simulink model "IFDA_5_2_Test1_Simulink"  (R2025b)
settings: Solver=VariableStepAuto  StartTime=0.0  StopTime=700  RelTol=1e-3
values from neighbouring files (symbols this model uses):
  lambda0 = zeros(6,1)    [IFDA_5_2_Test1.m]
  z0 = zeros(6,1)    [IFDA_5_2_Test1.m]
settings Model: Creator=ShuochengTian  LastModifiedBy=ShuochengTian
settings DataIOCC: ReturnWorkspaceOutputs=off

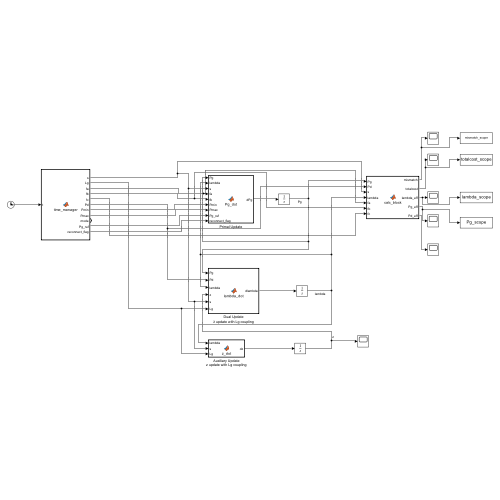
[thumbnail: Simulink's stored preview of the top-level diagram]
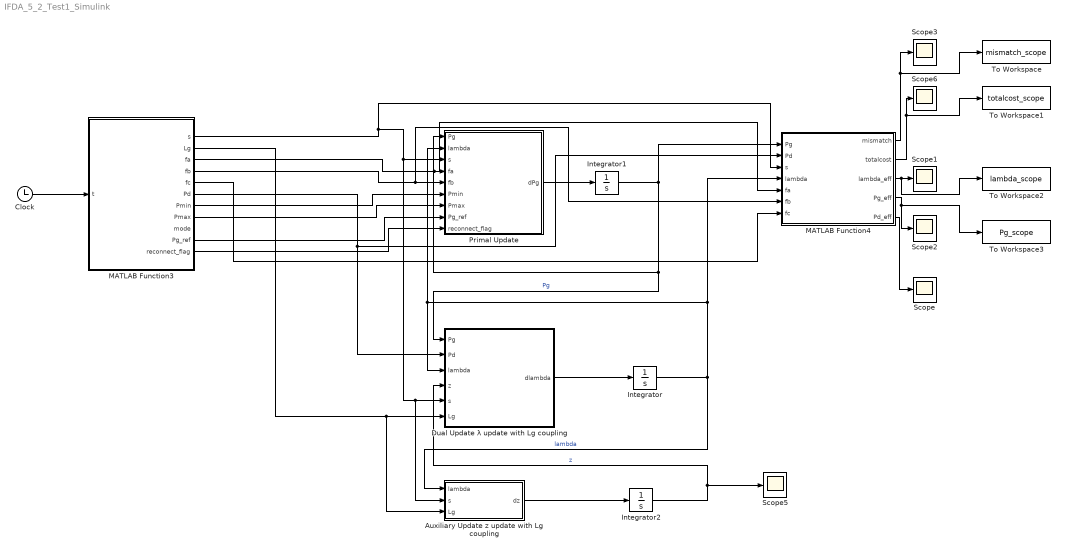
== system IFDA_5_2_Test1_Simulink ==
  Auxiliary Update z update with Lg coupling : MATLAB Function  TreatAsAtomicUnit=on
  Clock : Clock
  Dual Update λ update with Lg coupling : MATLAB Function  TreatAsAtomicUnit=on
  Integrator : Integrator  InitialCondition=lambda0
  Integrator1 : Integrator  InitialCondition=[0;0;0;0;0;0]
  Integrator2 : Integrator  InitialCondition=z0
  MATLAB Function3 : MATLAB Function  TreatAsAtomicUnit=on
  MATLAB Function4 : MATLAB Function  TreatAsAtomicUnit=on
  Primal Update : MATLAB Function  TreatAsAtomicUnit=on
  Scope{,1..3,5..6} (6 alike) : Scope
      Scope settings: ActiveDisplayYMinimum=-1  ActiveDisplayYMaximum=1
      Scope1 settings: ActiveDisplayYMinimum=-65.150992520934949  ActiveDisplayYMaximum=108.34326457907353
      Scope2 settings: ActiveDisplayYMinimum=-20.980945612997647  ActiveDisplayYMaximum=188.82851051697887  DataLoggingVariableName=Pg_scope
      Scope3 settings: ActiveDisplayYMinimum=-491.25638356925219  ActiveDisplayYMaximum=557.32192082133315  DataLoggingVariableName=ScopeData3
      Scope5 settings: ActiveDisplayYMinimum=-43.668129807631672  ActiveDisplayYMaximum=39.234905001957  DataLoggingVariableName=ScopeData5
      Scope6 settings: ActiveDisplayYMinimum=-1090.2784061772797  ActiveDisplayYMaximum=14121.754852896567  DataLoggingVariableName=ScopeData6
  To Workspace : ToWorkspace  VariableName=mismatch_scope  SaveFormat=Structure With Time  SampleTime=-1
  To Workspace1 : ToWorkspace  VariableName=totalcost_scope  SaveFormat=Structure With Time  SampleTime=-1
  To Workspace2 : ToWorkspace  VariableName=lambda_scope  SaveFormat=Structure With Time  SampleTime=-1
  To Workspace3 : ToWorkspace  VariableName=Pg_scope  SaveFormat=Structure With Time  SampleTime=-1
  wires:
  Integrator1/1 -> Primal Update/1(Pg), Dual Update λ update with Lg coupling/1(Pg), MATLAB Function4/1(Pg)  "Pg"
  Integrator2/1 -> Scope5/1, Dual Update λ update with Lg coupling/4(z)  "z"
  Auxiliary Update z update with Lg coupling/1(dz) -> Integrator2/1
  Integrator/1 -> MATLAB Function4/4(lambda), Dual Update λ update with Lg coupling/3(lambda), Primal Update/2(lambda), Auxiliary Update z update with Lg coupling/1(lambda)  "lambda"
  Primal Update/1(dPg) -> Integrator1/1
  MATLAB Function3/6(Pd) -> Dual Update λ update with Lg coupling/2(Pd), MATLAB Function4/2(Pd)
  Dual Update λ update with Lg coupling/1(dlambda) -> Integrator/1
  Clock/1 -> MATLAB Function3/1(t)
  MATLAB Function3/1(s) -> MATLAB Function4/3(s), Auxiliary Update z update with Lg coupling/2(s), Dual Update λ update with Lg coupling/5(s), Primal Update/3(s)
  MATLAB Function3/2(Lg) -> Dual Update λ update with Lg coupling/6(Lg), Auxiliary Update z update with Lg coupling/3(Lg)
  MATLAB Function3/3(fa) -> MATLAB Function4/5(fa), Primal Update/4(fa)
  MATLAB Function3/4(fb) -> Primal Update/5(fb), MATLAB Function4/6(fb)
  MATLAB Function3/7(Pmin) -> Primal Update/6(Pmin)
  MATLAB Function3/8(Pmax) -> Primal Update/7(Pmax)
  MATLAB Function3/10(Pg_ref) -> Primal Update/8(Pg_ref)
  MATLAB Function3/11(reconnect_flag) -> Primal Update/9(reconnect_flag)
  MATLAB Function4/1(mismatch) -> To Workspace/1, Scope3/1
  MATLAB Function4/4(Pg_eff) -> Scope2/1, To Workspace3/1
  MATLAB Function4/2(totalcost) -> To Workspace1/1, Scope6/1
  MATLAB Function3/5(fc) -> MATLAB Function4/7(fc)
  MATLAB Function4/5(Pd_eff) -> Scope/1
  MATLAB Function4/3(lambda_eff) -> To Workspace2/1, Scope1/1

== matlab function IFDA_5_2_Test1_Simulink/Dual Update λ update with Lg coupling ==
  data: Pg input; Pd input; dlambda output; lambda input; z input; s input; Lg input
function dlambda = lambda_dot(Pg, Pd, lambda, z, s, Lg)

n = 6;
dlambda = zeros(n,1);
%实际参与系统供需平衡的发电功率

Pg_eff = s .* Pg;
Pd_eff = s .* Pd;

%按资源分配算法计算原始

dlambda_raw = -Lg * lambda - Lg * z + (Pd_eff - Pg_eff);
%dlambda = dlambda_raw;

%对离线节点可选择冻结
for i = 1:n
   if s(i) == 0
       dlambda(i) = 0;
   else
       dlambda(i) = dlambda_raw(i);
   end
end

== matlab function IFDA_5_2_Test1_Simulink/Primal Update ==
  data: Pg input; lambda input; s input; fa input; fb input; Pmin input; Pmax input; Pg_ref input; dPg output; reconnect_flag input
function dPg = Pg_dot(Pg, lambda, s, fa, fb, Pmin, Pmax, Pg_ref, reconnect_flag)

n = 6;
dPg = zeros(n,1);
kr = 50;

for i = 1:n
    %% 若机组离线，直接冻结
    if s(i) == 0
        dPg(i) = 0;
        
    %% 若机组处于恢复过渡阶段
    elseif reconnect_flag(i) == 1
        v_i = kr * (Pg_ref(i) - Pg(i));
        if (Pg(i) <= Pmin(i)) && (v_i < 0)
            dPg(i) = 0;
        elseif (Pg(i) >= Pmax(i)) && (v_i > 0)
            dPg(i) = 0;
        else
            dPg(i) = v_i;
        end
        
    %% 正常在线运行：按原投影动态
    else
        
        grad_i = 2*fa(i)*Pg(i) + fb(i);
        
        
        v_i = -grad_i + lambda(i);
        
        if (Pg(i) <= Pmin(i)) && (v_i < 0)
            dPg(i) = 0;
        elseif (Pg(i) >= Pmax(i)) && (v_i > 0)
            dPg(i) = 0;
        else
            dPg(i) = v_i;
        end
    end
end

== matlab function IFDA_5_2_Test1_Simulink/Auxiliary Update z update with Lg coupling ==
  data: lambda input; dz output; s input; Lg input
function dz = z_dot(lambda, s, Lg)

n = 6;
dz = zeros(n,1);


% 先计算原始动态
dz_raw = Lg * lambda;
%dz = dz_raw;


% 对离线节点冻结
for i = 1:n
    if s(i) == 0
        dz(i) = 0;
    else
        dz(i) = dz_raw(i);
    end
end

== matlab function IFDA_5_2_Test1_Simulink/MATLAB Function3 ==
  data: t input; s output; Lg output; fa output; fb output; fc output; Pd output; Pmin output; Pmax output; mode output; Pg_ref output; reconnect_flag output
function [s,Lg,fa,fb,fc,Pd,Pmin,Pmax,mode,Pg_ref,reconnect_flag] = time_manager(t)
%% 断开前的旧配置
a_pre = [0.0100; 0.0250; 0.0200; 0.0090; 0.0180; 0.0340];

b_pre = [10.5;   12.0;   15.0;   11.5;   13.0;   9.5];

c_pre = [20; 25; 30; 22; 28; 18];

Pd_pre = [90; 80; 70; 85; 60; 55];

Pmin_pre = [20; 25; 15; 30; 18; 12];

Pmax_pre = [180; 200; 160; 220; 170; 150];

%% 恢复后的新配置
a_post = a_pre;
b_post = b_pre;
c_post = c_pre;
Pd_post = Pd_pre;
Pmin_post = Pmin_pre;
Pmax_post = Pmax_pre;

Pd_post(1)   = 28;
Pmin_post(1) = 15;
Pmax_post(1) = 60;

%% 原始通信图

L_normal = [ 2 -1  0  0  0 -1;
            -1  3 -1  0  -1  0;
            0 -1  3 -1  0  -1;
            0  0 -1  2 -1  0;
            0  -1  0 -1  3 -1;
     -      1  0  -1  0 -1  3];


%% 断开时的通信图

L_off = [ 0 0  0  0  0 0;
        0  2 -1  0  -1  0;
        0 -1  3 -1  0  -1;
        0  0 -1  2 -1  0;
        0  -1  0 -1  3 -1;
        0  0  -1  0 -1  2];


%% 恢复后的通信图

L_recover = L_normal;


%% 时间分段
if t < 300
    
    %正常运行
    s = ones(6,1);
    Lg = L_normal;

    fa = a_pre;
    fb = b_pre;
    fc = c_pre;
    Pd = Pd_pre;
    Pmin = Pmin_pre;
    Pmax = Pmax_pre;

    mode = 1;

    Pg_ref = zeros(6,1);
    reconnect_flag = zeros(6,1);

elseif t < 500
    
    %Pd保持原值不变（总需求不变）
    s = [0;1;1;1;1;1];
    Lg = L_off;

    fa = a_pre;
    fb = b_pre;
    fc = c_pre;
    Pd = Pd_pre;
    Pmin = Pmin_pre;
    Pmax = Pmax_pre;

    mode = 2;

    Pg_ref = zeros(6,1);
    reconnect_flag = zeros(6,1);

elseif t < 502
    %发电机重新接入，但不希望直接按断开前旧Pg值运行

    s = ones(6,1);
    Lg = L_recover;

    fa = a_post;
    fb = b_post;
    fc = c_post;
    Pd = Pd_post;
    Pmin = Pmin_post;
    Pmax = Pmax_post;

    mode = 3;

    %恢复过渡
    reconnect_flag = [1;0;0;0;0;0];

    %发电机恢复时参考功率
    %取新上下界中点，保证满足新约束
    Pg_ref = zeros(6,1);
    Pg_ref(1) = 0.5 * (Pmin_post(1) + Pmax_post(1));

else
    %恢复后正常运行
    s = ones(6,1);
    Lg = L_recover;

    fa = a_post;
    fb = b_post;
    fc = c_post;
    Pd = Pd_post;
    Pmin = Pmin_post;
    Pmax = Pmax_post;

    mode = 4;

    Pg_ref = zeros(6,1);
    reconnect_flag = zeros(6,1);
end
end

== matlab function IFDA_5_2_Test1_Simulink/MATLAB Function4 ==
  data: Pg input; mismatch output; totalcost output; lambda_eff output; Pd input; s input; Pg_eff output; Pd_eff output; lambda input; fa input; fb input; fc input
function [mismatch, totalcost, lambda_eff, Pg_eff, Pd_eff] = calc_block(Pg, Pd, s, lambda, fa, fb, fc)


Pg_eff = s .* Pg;
Pd_eff = s .* Pd;

fa_eff = s .* fa;
fb_eff = s .* fb;
fc_eff = s .* fc;

mismatch = sum(Pg_eff) - sum(Pd_eff);

n = 6;
cost = zeros(n,1);
for i = 1:n
    cost(i) = fa_eff(i)*Pg_eff(i)^2 + fb_eff(i) * Pg_eff(i) + fc_eff(i);
end
totalcost = sum(cost);

lambda_eff = s .* lambda;
end
